simulink model "EO_IR_Sensor_Manager"  (R2026a)
settings: Solver=FixedStepDiscrete  StopTime=120  FixedStep=0.05
settings Model: Creator=Avatec  LastModifiedBy=Avatec

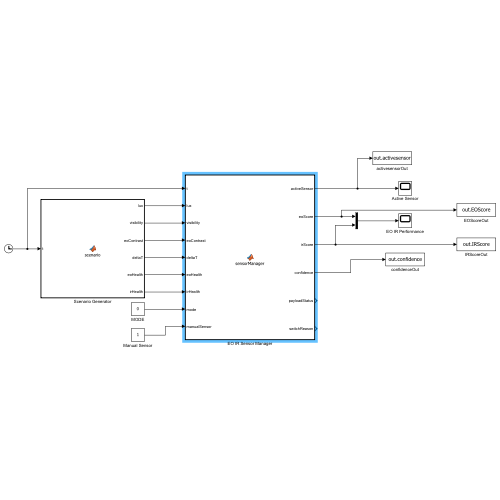
[thumbnail: Simulink's stored preview of the top-level diagram]
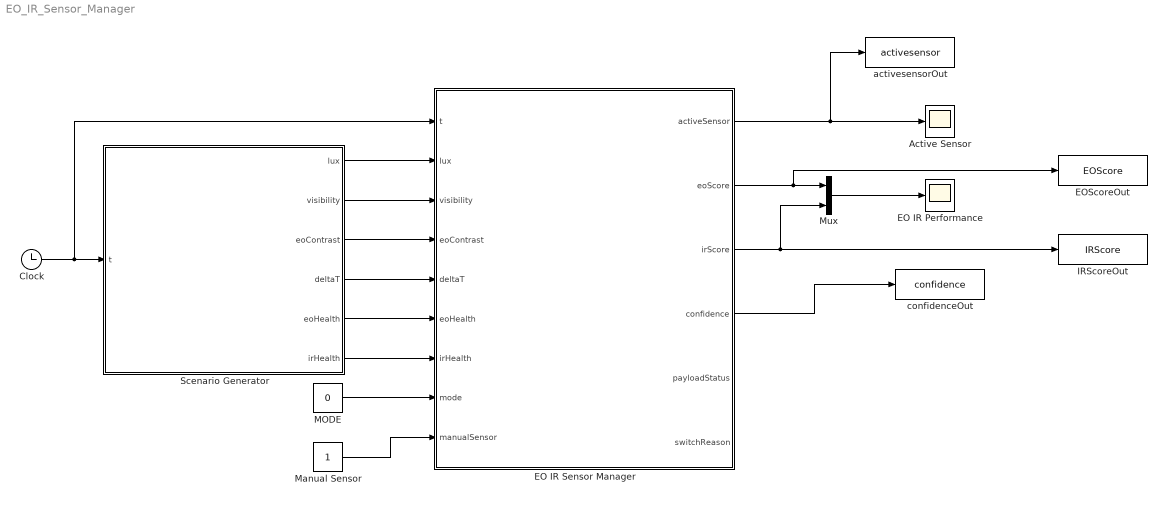
== system EO_IR_Sensor_Manager ==
  Active Sensor : Scope
      settings: ActiveDisplayYMinimum=-0.9771153722645658  ActiveDisplayYMaximum=4.0737650945561565
  Clock : Clock
  EO IR Performance : Scope
      settings: ActiveDisplayYMinimum=1.7792893969156722  ActiveDisplayYMaximum=124.98117919695903
  EO IR Sensor Manager : MATLAB Function  TreatAsAtomicUnit=on
  EOScoreOut : ToWorkspace  VariableName=EOScore  SaveFormat=Timeseries  SampleTime=-1
  IRScoreOut : ToWorkspace  VariableName=IRScore  SaveFormat=Timeseries  SampleTime=-1
  MODE : Constant  Value=0
  Manual Sensor : Constant
  Mux : Mux  Inputs=2
  Scenario Generator : MATLAB Function  TreatAsAtomicUnit=on
  activesensorOut : ToWorkspace  VariableName=activesensor  SaveFormat=Timeseries  SampleTime=-1
  confidenceOut : ToWorkspace  VariableName=confidence  SaveFormat=Timeseries  SampleTime=-1
  wires:
  Clock/1 -> EO IR Sensor Manager/1(t), Scenario Generator/1(t)
  Scenario Generator/1(lux) -> EO IR Sensor Manager/2(lux)
  Scenario Generator/2(visibility) -> EO IR Sensor Manager/3(visibility)
  Scenario Generator/3(eoContrast) -> EO IR Sensor Manager/4(eoContrast)
  Scenario Generator/4(deltaT) -> EO IR Sensor Manager/5(deltaT)
  Scenario Generator/5(eoHealth) -> EO IR Sensor Manager/6(eoHealth)
  Scenario Generator/6(irHealth) -> EO IR Sensor Manager/7(irHealth)
  MODE/1 -> EO IR Sensor Manager/8(mode)
  Manual Sensor/1 -> EO IR Sensor Manager/9(manualSensor)
  EO IR Sensor Manager/2(eoScore) -> EOScoreOut/1, Mux/1
  EO IR Sensor Manager/3(irScore) -> IRScoreOut/1, Mux/2
  Mux/1 -> EO IR Performance/1
  EO IR Sensor Manager/1(activeSensor) -> activesensorOut/1, Active Sensor/1
  EO IR Sensor Manager/4(confidence) -> confidenceOut/1

== matlab function EO_IR_Sensor_Manager/EO IR Sensor Manager ==
  data: t input; activeSensor output; lux input; visibility input; eoContrast input; deltaT input; eoHealth input; irHealth input; mode input; manualSensor input; eoScore output; irScore output; confidence output; payloadStatus output; switchReason output
function [activeSensor, eoScore, irScore, confidence, ...
          payloadStatus, switchReason] = ...
          sensorManager(t, lux, visibility, eoContrast, ...
                        deltaT, eoHealth, irHealth, ...
                        mode, manualSensor)

% ============================================
% ADAPTIVE EO / IR SENSOR MANAGER
% ============================================

persistent currentSensor
persistent candidateSensor
persistent candidateStart
persistent lastSwitchReason

% --------------------------------------------
% INITIALIZATION
% --------------------------------------------

if isempty(currentSensor)

    currentSensor = 1;       % Start with EO
    candidateSensor = 0;
    candidateStart = 0;
    lastSwitchReason = 0;

end


% ============================================
% PARAMETERS
% ============================================

hysteresis = 10;
confirmationTime = 2;


% ============================================
% EO PERFORMANCE MODEL
% ============================================

% Illumination normalization
L = log10(max(lux,0) + 1) / log10(10001);

L = min(max(L,0),1);


% Visibility normalization
V = visibility / 10;

V = min(max(V,0),1);


% EO contrast normalization
C = min(max(eoContrast,0),1);


% EO performance score
eoScore = 100 * ...
    (0.50*L + ...
     0.30*V + ...
     0.20*C);


% ============================================
% IR PERFORMANCE MODEL
% ============================================

% Thermal contrast normalization
T = abs(deltaT) / 10;

T = min(max(T,0),1);


% IR performance score
irScore = 100 * ...
    (0.70*T + ...
     0.30*V);


% ============================================
% MANUAL MODE
% ============================================

if mode == 1

    if manualSensor == 1 && eoHealth == 1

        currentSensor = 1;
        lastSwitchReason = 6;

    elseif manualSensor == 2 && irHealth == 1

        currentSensor = 2;
        lastSwitchReason = 6;

    elseif eoHealth == 1

        currentSensor = 1;

    elseif irHealth == 1

        currentSensor = 2;

    else

        currentSensor = 0;
        lastSwitchReason = 5;

    end

    candidateSensor = 0;
    candidateStart = t;


% ============================================
% AUTO MODE
% ============================================

else

    % ----------------------------------------
    % BOTH SENSORS FAILED
    % ----------------------------------------

    if eoHealth == 0 && irHealth == 0

        currentSensor = 0;

        candidateSensor = 0;
        candidateStart = t;

        lastSwitchReason = 5;


    % ----------------------------------------
    % EO FAILED
    % ----------------------------------------

    elseif eoHealth == 0 && irHealth == 1

        if currentSensor ~= 2

            lastSwitchReason = 3;

        end

        currentSensor = 2;

        candidateSensor = 0;
        candidateStart = t;


    % ----------------------------------------
    % IR FAILED
    % ----------------------------------------

    elseif irHealth == 0 && eoHealth == 1

        if currentSensor ~= 1

            lastSwitchReason = 4;

        end

        currentSensor = 1;

        candidateSensor = 0;
        candidateStart = t;


    % ----------------------------------------
    % BOTH SENSORS HEALTHY
    % ----------------------------------------

    else

        % ====================================
        % EO ACTIVE
        % ====================================

        if currentSensor == 1

            % Is IR significantly better?
            if irScore > eoScore + hysteresis

                if candidateSensor ~= 2

                    candidateSensor = 2;
                    candidateStart = t;

                else

                    % Has IR remained better
                    % for long enough?
                    if (t - candidateStart) >= ...
                            confirmationTime

                        currentSensor = 2;

                        candidateSensor = 0;

                        lastSwitchReason = 1;

                    end
                end

            else

                % Cancel pending switch
                candidateSensor = 0;
                candidateStart = t;

            end


        % ====================================
        % IR ACTIVE
        % ====================================

        elseif currentSensor == 2

            % Is EO significantly better?
            if eoScore > irScore + hysteresis

                if candidateSensor ~= 1

                    candidateSensor = 1;
                    candidateStart = t;

                else

                    if (t - candidateStart) >= ...
                            confirmationTime

                        currentSensor = 1;

                        candidateSensor = 0;

                        lastSwitchReason = 2;

                    end
                end

            else

                candidateSensor = 0;
                candidateStart = t;

            end


        % ====================================
        % RECOVERY FROM FAULT
        % ====================================

        else

            if eoScore >= irScore

                currentSensor = 1;

            else

                currentSensor = 2;

            end

        end
    end
end


% ============================================
% OUTPUTS
% ============================================

activeSensor = currentSensor;

switchReason = lastSwitchReason;


% --------------------------------------------
% CONFIDENCE
% --------------------------------------------

if currentSensor == 1

    confidence = eoScore;

elseif currentSensor == 2

    confidence = irScore;

else

    confidence = 0;

end


% --------------------------------------------
% PAYLOAD STATUS
%
% 0 = FAULT
% 1 = OPERATIONAL
% 2 = DEGRADED
% --------------------------------------------

if currentSensor == 0

    payloadStatus = 0;

elseif confidence >= 50

    payloadStatus = 1;

else

    payloadStatus = 2;

end

== matlab function EO_IR_Sensor_Manager/Scenario Generator ==
  data: t input; lux output; visibility output; eoContrast output; deltaT output; eoHealth output; irHealth output
function [lux, visibility, eoContrast, deltaT, ...
    eoHealth, irHealth] = scenario(t)

% ============================================
% ADAPTIVE EO/IR TEST SCENARIO
% ============================================

% --------------------------------------------
% AMBIENT ILLUMINATION
% Day -> sunset -> night
% --------------------------------------------

lux = 50000 * exp(-0.09*t) + 1;


% --------------------------------------------
% VISIBILITY
% Slowly changing atmospheric visibility
% --------------------------------------------

visibility = 12 ...
    - 0.035*t ...
    + 1.0*sin(0.07*t);

visibility = min(max(visibility,2),15);


% --------------------------------------------
% EO SCENE CONTRAST
% Slowly changing visible scene contrast
% --------------------------------------------

eoContrast = 0.78 ...
    - 0.0015*t ...
    + 0.05*sin(0.10*t);

eoContrast = min(max(eoContrast,0.30),1);


% --------------------------------------------
% THERMAL CONTRAST
%
% First increases during night conditions.
% Then decreases due to thermal crossover.
% --------------------------------------------

riseTerm = 5 / ...
    (1 + exp(-(t-55)/6));

fallTerm = 8 / ...
    (1 + exp(-(t-90)/4));

deltaT = 3 + riseTerm - fallTerm;

deltaT = max(deltaT,0.5);


% --------------------------------------------
% SENSOR HEALTH
% --------------------------------------------

eoHealth = 1;
irHealth = 1;

% EO sensor fault
if t >= 105
    eoHealth = 0;
end

% IR sensor fault
if t >= 114
    irHealth = 0;
end
